simulink model "lab2a"  (Simulink 7.3)
settings: Solver=FixedStepDiscrete  StartTime=0.0  StopTime=10  FixedStep=sampletime  RelTol=1e-3
libraries: dspsrcs4 x4, dspbuff3 x3, dspsnks4 x1
settings Model: Creator=rtadm  LastModifiedBy=freli005
settings DataIOCC: LimitDataPoints=off
settings OptimizationCC: BooleanDataType=off
settings DebuggingCC: SaveWithParameterizedLinksMsg=none  SignalResolutionControl=TryResolveAllWithWarning  SolverPrmCheckMsg=none  MultiTaskDSMMsg=warning  MultiTaskCondExecSysMsg=none  StrictBusMsg=None
settings HardwareCC: TargetUnknown=on
settings RTWCC: IncludeERTFirstTime=on

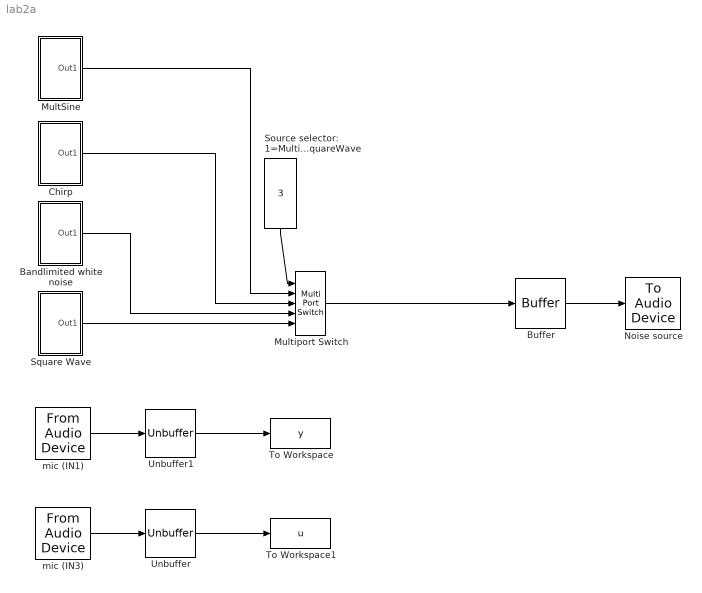
== system lab2a ==
  Bandlimited white noise : Subsystem
  Buffer : dspbuff3/Buffer  N=64  V=0  ic=0
  Chirp : Subsystem
  MultSine : Subsystem
  Multiport Switch : MultiPortSwitch  Inputs=4  SaturateOnIntegerOverflow=on  InputSameDT=on
  Noise source : dspsnks4/To Audio Device  DialogController=dspDDGCreate  DialogControllerArgs=DataTag1  deviceName=5,6-INCA 88 Stereo Wave  inheritSampleRate=on  sampleRate=44100  deviceDatatype=Determine from input data type  autoBufferSize=on  bufferSize=4096  queueDuration=0.1
  Source selector: 1=MultiSine 2=Chirp 3=White noise 4=SquareWave : Constant  Value=3
  Square Wave : Subsystem
  To Workspace : ToWorkspace  VariableName=y  SampleTime=sampletime  SaveFormat=Array
  To Workspace1 : ToWorkspace  VariableName=u  SampleTime=sampletime  SaveFormat=Array
  Unbuffer : dspbuff3/Unbuffer  ic=0
  Unbuffer1 : dspbuff3/Unbuffer  ic=0
  mic (IN1) : dspsrcs4/From Audio Device  DialogController=dspDDGCreate  DialogControllerArgs=DataTag2  deviceName=1,2-INCA 88 Stereo Wave  numChannels=1  sampleRate=11025  deviceDatatype=Determine from output data type  autoBufferSize=on  bufferSize=4096  queueDuration=3  frameSize=64  outputDatatype=double
  mic (IN3) : dspsrcs4/From Audio Device  DialogController=dspDDGCreate  DialogControllerArgs=DataTag3  deviceName=3,4-INCA 88 Stereo Wave  numChannels=1  sampleRate=11025  deviceDatatype=Determine from output data type  autoBufferSize=on  bufferSize=4096  queueDuration=3  frameSize=64  outputDatatype=double
  wires:
  mic (IN3)/1 -> Unbuffer/1
  Source selector: 1=MultiSine 2=Chirp 3=White noise 4=SquareWave/1 -> Multiport Switch/1
  Chirp/1(Out1) -> Multiport Switch/3
  Square Wave/1(Out1) -> Multiport Switch/5
  Multiport Switch/1 -> Buffer/1
  Unbuffer/1 -> To Workspace1/1
  Bandlimited white noise/1(Out1) -> Multiport Switch/4
  MultSine/1(Out1) -> Multiport Switch/2
  mic (IN1)/1 -> Unbuffer1/1
  Unbuffer1/1 -> To Workspace/1
  Buffer/1 -> Noise source/1

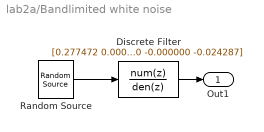
== system lab2a/Bandlimited white noise ==
  Discrete Filter : DiscreteFilter  Numerator=[0.277472 0.000000 -1.387362 0.000000 2.774724 0.000000 -2.774724 0.000000 1.387362 0.000000 -0.277472]*0.3  Denominator=[1.000000 -0.000000 -2.547368 0.000000 2.994845 -0.000000 -1.778046 0.000000 0.534570 -0.000000 -0.024287]  SampleTime=sampletime
  Random Source : dspsrcs4/Random Source  SrcType=Gaussian  NormMethod=Ziggurat  CltLength=12  MinVal=-1  MaxVal=1  MeanVal=0  VarVal=1  RepMode=Specify seed  rawSeed=1  IsInherit=off  SampMode=Discrete  SampTime=sampletime  SampFrame=1  DataType=Double  OutComplex=Real
  Out1 : Outport
  wires:
  Discrete Filter/1 -> Out1/1
  Random Source/1 -> Discrete Filter/1

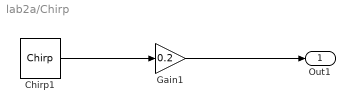
== system lab2a/Chirp ==
  Chirp1 : dspsrcs4/Chirp  sweep=Linear  mode=Bidirectional  f0=600  f1=800  t1=1  Tsweep=10  phase=0  Ts=sampletime  spf=1  datatype=Double
  Gain1 : Gain  Gain=0.2  SaturateOnIntegerOverflow=on  OutDataTypeStr=Inherit: Same as input  ParamDataTypeStr=Inherit: Same as input
  Out1 : Outport
  wires:
  Gain1/1 -> Out1/1
  Chirp1/1 -> Gain1/1

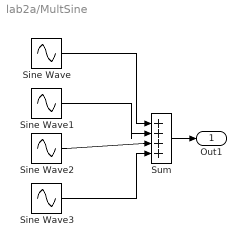
== system lab2a/MultSine ==
  Sine Wave : Sin  Amplitude=.1  Bias=0  Frequency=2*2400  Phase=0  Samples=10  SampleTime=sampletime  Offset=0
  Sine Wave1 : Sin  Amplitude=.1  Bias=0  Frequency=2*3000  Phase=0  Samples=10  SampleTime=sampletime  Offset=0
  Sine Wave2 : Sin  Amplitude=.1  Bias=0  Frequency=2*3600  Phase=0  Samples=10  SampleTime=sampletime  Offset=0
  Sine Wave3 : Sin  Amplitude=.1  Bias=0  Frequency=2*4200  Phase=0  Samples=10  SampleTime=sampletime  Offset=0
  Sum : Sum  Inputs=|++++  SaturateOnIntegerOverflow=on  InputSameDT=on  OutDataTypeStr=Inherit: Same as first input
  Out1 : Outport
  wires:
  Sine Wave/1 -> Sum/1
  Sine Wave1/1 -> Sum/2
  Sine Wave2/1 -> Sum/3
  Sine Wave3/1 -> Sum/4
  Sum/1 -> Out1/1

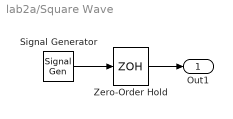
== system lab2a/Square Wave ==
  Signal Generator : SignalGenerator  WaveForm=square  Amplitude=.1  Frequency=100
  Zero-Order Hold : ZeroOrderHold  SampleTime=sampletime
  Out1 : Outport
  wires:
  Zero-Order Hold/1 -> Out1/1
  Signal Generator/1 -> Zero-Order Hold/1
